simulink model "Multicopter_Testbed"  (R2012b)
settings: Solver=FixedStepDiscrete  SolverMode=SingleTasking  StartTime=0.0  StopTime=inf  FixedStep=Sampletime.Sim  MaxStep=0.005  MinStep=0.0001  RelTol=1e-5
PreLoadFcn:
  | addpath([cd filesep 'Multicopter_Simulation_Data'])
  | initMulticopterSimulationBus;
  | initOveroControlBus;
  | initMulticopterSimulation;
undefined symbols (not defined in the file): Airframe_Pelican, DiscIntNeverNeededParam, Environment_Earth, gcbh, quat_fr_euler, rad, Sampletime, Sensor_Autopilot, vrmfunc
(part 2 of 3)

== system Multicopter_Testbed/Ground_Control/Extended_Debug_Demux/Compare To Constant4 ==
  u : Inport
  Compare : RelationalOperator  Operator===  OutDataTypeStr=fixdt(0, 8)  ZeroCross=off  InputSameDT=on
  Constant : Constant  DisableCoverage=on  Value=const  OutDataTypeStr=Inherit: Inherit via back propagation
  y : Outport
  wires:
  u/1 -> Compare/1
  Constant/1 -> Compare/2
  Compare/1 -> y/1

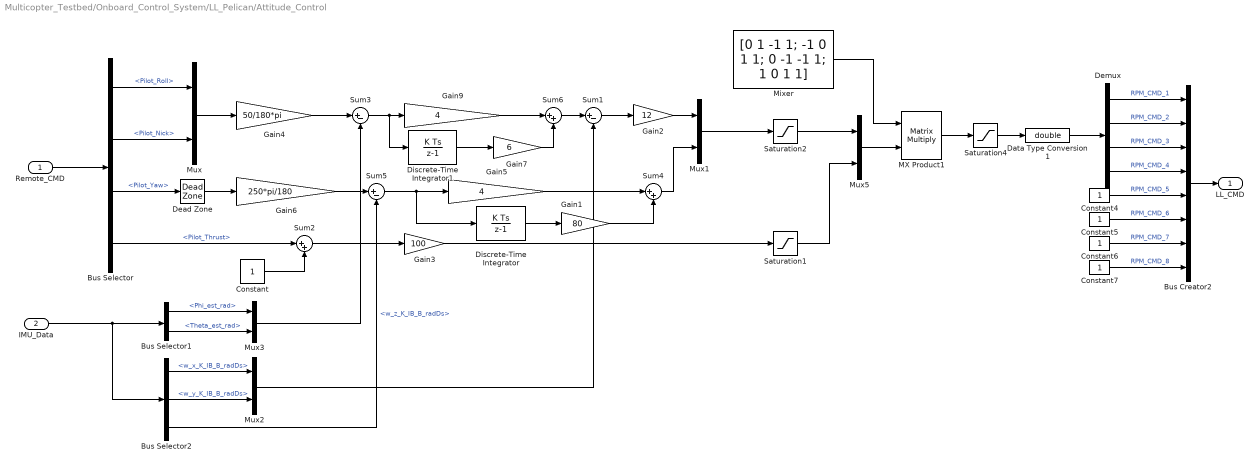
== system Multicopter_Testbed/Onboard_Control_System/LL_Pelican/Attitude_Control ==
  Remote_CMD : Inport
  IMU_Data : Inport  Port=2
  Bus Creator2 : BusCreator  Inputs=8
  Bus Selector : BusSelector  OutputSignals=Pilot_Roll,Pilot_Nick,Pilot_Yaw,Pilot_Thrust
  Bus Selector1 : BusSelector  OutputSignals=Phi_est_rad,Theta_est_rad
  Bus Selector2 : BusSelector  OutputSignals=w_x_K_IB_B_radDs,w_y_K_IB_B_radDs,w_z_K_IB_B_radDs
  Constant : Constant  OutDataTypeStr=single
  Constant{4..7} (4 alike) : Constant
  Data Type Conversion1 : DataTypeConversion  OutDataTypeStr=double
  Dead Zone : DeadZone  LowerValue=-0.1  UpperValue=0.1  SaturateOnIntegerOverflow=on
  Demux : Demux
  Discrete-Time Integrator : DiscreteIntegrator  SampleTime=-1  LimitOutput=on  UpperSaturationLimit=30/180*pi  LowerSaturationLimit=-30/180*pi  ICPrevOutput=DiscIntNeverNeededParam  ICPrevScaledInput=DiscIntNeverNeededParam
  Discrete-Time Integrator1 : DiscreteIntegrator  SampleTime=-1  LimitOutput=on  UpperSaturationLimit=5/180*pi  LowerSaturationLimit=-5/180*pi  ICPrevOutput=DiscIntNeverNeededParam  ICPrevScaledInput=DiscIntNeverNeededParam
  Gain1 : Gain  Gain=80
  Gain2 : Gain  Gain=12
  Gain3 : Gain  Gain=100
  Gain4 : Gain  Gain=50/180*pi
  Gain5 : Gain  Gain=4
  Gain6 : Gain  Gain=250*pi/180
  Gain7 : Gain  Gain=6
  Gain9 : Gain  Gain=4
  MX Product1 : Product  Multiplication=Matrix(*)  OutDataTypeStr=double  RndMeth=Simplest
  Mixer : Constant  Value=|  VectorParams1D=off  OutDataTypeStr=single
      | [0 1 -1 1; -1 0 1 1; 0 -1 -1 1;
      | 1 0 1 1]
  Mux{,1..3,5} (5 alike) : Mux  Inputs=2
  Saturation1 : Saturate  UpperLimit=170  LowerLimit=1
  Saturation2 : Saturate  UpperLimit=100  LowerLimit=-100
  Saturation4 : Saturate  UpperLimit=200  LowerLimit=1  OutDataTypeStr=int16
  Sum1 : Sum  Inputs=|+-
  Sum2 : Sum  Inputs=|++
  Sum3 : Sum  Inputs=|+-
  Sum4 : Sum  Inputs=|++
  Sum5 : Sum  Inputs=|+-
  Sum6 : Sum  Inputs=|++
  LL_CMD : Outport
  wires:
  Gain7/1 -> Sum6/2
  Discrete-Time Integrator1/1 -> Gain7/1
  Sum6/1 -> Sum1/1
  Data Type Conversion1/1 -> Demux/1
  Bus Creator2/1 -> LL_CMD/1
  Demux/4 -> Bus Creator2/4  "RPM_CMD_4"
  Demux/3 -> Bus Creator2/3  "RPM_CMD_3"
  Demux/2 -> Bus Creator2/2  "RPM_CMD_2"
  Demux/1 -> Bus Creator2/1  "RPM_CMD_1"
  Constant7/1 -> Bus Creator2/8  "RPM_CMD_8"
  Constant6/1 -> Bus Creator2/7  "RPM_CMD_7"
  Constant5/1 -> Bus Creator2/6  "RPM_CMD_6"
  Constant4/1 -> Bus Creator2/5  "RPM_CMD_5"
  Saturation4/1 -> Data Type Conversion1/1
  IMU_Data/1 -> Bus Selector2/1, Bus Selector1/1
  Gain4/1 -> Sum3/1
  Bus Selector1/2 -> Mux3/2  "<Theta_est_rad>"
  Bus Selector1/1 -> Mux3/1  "<Phi_est_rad>"
  Constant/1 -> Sum2/2
  Sum2/1 -> Gain3/1
  Saturation2/1 -> Mux5/1
  Saturation1/1 -> Mux5/2
  Mixer/1 -> MX Product1/1
  Mux5/1 -> MX Product1/2
  MX Product1/1 -> Saturation4/1
  Mux1/1 -> Saturation2/1
  Gain3/1 -> Saturation1/1
  Bus Selector/3 -> Dead Zone/1  "<Pilot_Yaw>"
  Bus Selector/2 -> Mux/2  "<Pilot_Nick>"
  Bus Selector/1 -> Mux/1  "<Pilot_Roll>"
  Remote_CMD/1 -> Bus Selector/1
  Mux3/1 -> Sum3/2
  Bus Selector2/3 -> Sum5/2  "<w_z_K_IB_B_radDs>"
  Mux/1 -> Gain4/1
  Bus Selector2/2 -> Mux2/2  "<w_y_K_IB_B_radDs>"
  Bus Selector2/1 -> Mux2/1  "<w_x_K_IB_B_radDs>"
  Sum3/1 -> Gain9/1, Discrete-Time Integrator1/1
  Bus Selector/4 -> Sum2/1  "<Pilot_Thrust>"
  Gain2/1 -> Mux1/1
  Sum5/1 -> Gain5/1, Discrete-Time Integrator/1
  Gain6/1 -> Sum5/1
  Sum1/1 -> Gain2/1
  Gain9/1 -> Sum6/1
  Mux2/1 -> Sum1/2
  Dead Zone/1 -> Gain6/1
  Discrete-Time Integrator/1 -> Gain1/1
  Gain1/1 -> Sum4/2
  Gain5/1 -> Sum4/1
  Sum4/1 -> Mux1/2

== system Multicopter_Testbed/Onboard_Control_System/LL_Pelican/Compare To Zero ==
  u : Inport
  Compare : RelationalOperator  Operator=>  OutDataTypeStr=fixdt(0, 8)  InputSameDT=on
  Constant : Constant  DisableCoverage=on  Value=0  OutDataTypeStr=Inherit: Inherit via back propagation  PreserveConstantTs=on
  y : Outport
  wires:
  Constant/1 -> Compare/2
  u/1 -> Compare/1
  Compare/1 -> y/1

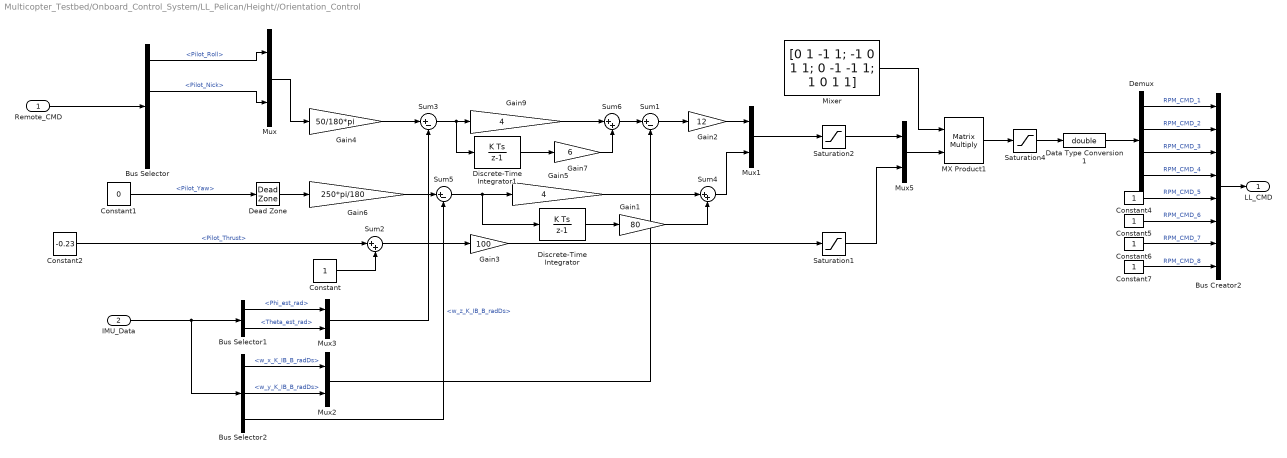
== system Multicopter_Testbed/Onboard_Control_System/LL_Pelican/Height//Orientation_Control ==
  Remote_CMD : Inport
  IMU_Data : Inport  Port=2
  Bus Creator2 : BusCreator  Inputs=8
  Bus Selector : BusSelector  OutputSignals=Pilot_Roll,Pilot_Nick,Pilot_Yaw,Pilot_Thrust
  Bus Selector1 : BusSelector  OutputSignals=Phi_est_rad,Theta_est_rad
  Bus Selector2 : BusSelector  OutputSignals=w_x_K_IB_B_radDs,w_y_K_IB_B_radDs,w_z_K_IB_B_radDs
  Constant : Constant  OutDataTypeStr=single
  Constant1 : Constant  Value=0  OutDataTypeStr=single
  Constant2 : Constant  Value=-0.23  OutDataTypeStr=single
  Constant{4..7} (4 alike) : Constant
  Data Type Conversion1 : DataTypeConversion  OutDataTypeStr=double
  Dead Zone : DeadZone  LowerValue=-0.1  UpperValue=0.1  SaturateOnIntegerOverflow=on
  Demux : Demux
  Discrete-Time Integrator : DiscreteIntegrator  SampleTime=-1  LimitOutput=on  UpperSaturationLimit=30/180*pi  LowerSaturationLimit=-30/180*pi  ICPrevOutput=DiscIntNeverNeededParam  ICPrevScaledInput=DiscIntNeverNeededParam
  Discrete-Time Integrator1 : DiscreteIntegrator  SampleTime=-1  LimitOutput=on  UpperSaturationLimit=5/180*pi  LowerSaturationLimit=-5/180*pi  ICPrevOutput=DiscIntNeverNeededParam  ICPrevScaledInput=DiscIntNeverNeededParam
  Gain1 : Gain  Gain=80
  Gain2 : Gain  Gain=12
  Gain3 : Gain  Gain=100
  Gain4 : Gain  Gain=50/180*pi
  Gain5 : Gain  Gain=4
  Gain6 : Gain  Gain=250*pi/180
  Gain7 : Gain  Gain=6
  Gain9 : Gain  Gain=4
  MX Product1 : Product  Multiplication=Matrix(*)  OutDataTypeStr=double  RndMeth=Simplest
  Mixer : Constant  Value=|  VectorParams1D=off  OutDataTypeStr=single
      | [0 1 -1 1; -1 0 1 1; 0 -1 -1 1;
      | 1 0 1 1]
  Mux{,1..3,5} (5 alike) : Mux  Inputs=2
  Saturation1 : Saturate  UpperLimit=170  LowerLimit=1
  Saturation2 : Saturate  UpperLimit=100  LowerLimit=-100
  Saturation4 : Saturate  UpperLimit=200  LowerLimit=1  OutDataTypeStr=int16
  Sum1 : Sum  Inputs=|+-
  Sum2 : Sum  Inputs=|++
  Sum3 : Sum  Inputs=|+-
  Sum4 : Sum  Inputs=|++
  Sum5 : Sum  Inputs=|+-
  Sum6 : Sum  Inputs=|++
  LL_CMD : Outport
  wires:
  Sum4/1 -> Mux1/2
  Gain5/1 -> Sum4/1
  Gain1/1 -> Sum4/2
  Discrete-Time Integrator/1 -> Gain1/1
  Dead Zone/1 -> Gain6/1
  Mux2/1 -> Sum1/2
  Gain9/1 -> Sum6/1
  Sum1/1 -> Gain2/1
  Gain6/1 -> Sum5/1
  Sum5/1 -> Discrete-Time Integrator/1, Gain5/1
  Gain2/1 -> Mux1/1
  Constant2/1 -> Sum2/1  "<Pilot_Thrust>"
  Sum3/1 -> Discrete-Time Integrator1/1, Gain9/1
  Bus Selector2/1 -> Mux2/1  "<w_x_K_IB_B_radDs>"
  Bus Selector2/2 -> Mux2/2  "<w_y_K_IB_B_radDs>"
  Mux/1 -> Gain4/1
  Bus Selector2/3 -> Sum5/2  "<w_z_K_IB_B_radDs>"
  Mux3/1 -> Sum3/2
  Remote_CMD/1 -> Bus Selector/1
  Bus Selector/1 -> Mux/1  "<Pilot_Roll>"
  Bus Selector/2 -> Mux/2  "<Pilot_Nick>"
  Constant1/1 -> Dead Zone/1  "<Pilot_Yaw>"
  Gain3/1 -> Saturation1/1
  Mux1/1 -> Saturation2/1
  MX Product1/1 -> Saturation4/1
  Mux5/1 -> MX Product1/2
  Mixer/1 -> MX Product1/1
  Saturation1/1 -> Mux5/2
  Saturation2/1 -> Mux5/1
  Sum2/1 -> Gain3/1
  Constant/1 -> Sum2/2
  Bus Selector1/1 -> Mux3/1  "<Phi_est_rad>"
  Bus Selector1/2 -> Mux3/2  "<Theta_est_rad>"
  Gain4/1 -> Sum3/1
  IMU_Data/1 -> Bus Selector1/1, Bus Selector2/1
  Saturation4/1 -> Data Type Conversion1/1
  Constant4/1 -> Bus Creator2/5  "RPM_CMD_5"
  Constant5/1 -> Bus Creator2/6  "RPM_CMD_6"
  Constant6/1 -> Bus Creator2/7  "RPM_CMD_7"
  Constant7/1 -> Bus Creator2/8  "RPM_CMD_8"
  Demux/1 -> Bus Creator2/1  "RPM_CMD_1"
  Demux/2 -> Bus Creator2/2  "RPM_CMD_2"
  Demux/3 -> Bus Creator2/3  "RPM_CMD_3"
  Demux/4 -> Bus Creator2/4  "RPM_CMD_4"
  Bus Creator2/1 -> LL_CMD/1
  Data Type Conversion1/1 -> Demux/1
  Sum6/1 -> Sum1/1
  Discrete-Time Integrator1/1 -> Gain7/1
  Gain7/1 -> Sum6/2

== system Multicopter_Testbed/Onboard_Control_System/LL_Signal_Processing/GPS_Signal_Processing ==
  Inputs : Inport  OutDataTypeStr=Bus: Sensor_Data_Bus
  Bus Creator1 : BusCreator  Inputs=16  OutDataTypeStr=Bus: FCS_GPS_Bus  NonVirtualBus=on
  Bus Selector : BusSelector  OutputSignals=GPS_Data.POS_lambda_WGS84,GPS_Data.POS_mue_WGS84,GPS_Data.POS_h_WGS84
  Bus Selector1 : BusSelector  OutputSignals=GPS_Data.VEL_x_E_O,GPS_Data.VEL_y_E_O
  Constant10 : Constant  Value=1696  OutDataTypeStr=int32
  Constant11 : Constant  Value=129600000  OutDataTypeStr=int32
  Constant12 : Constant  Value=6  OutDataTypeStr=int32
  Constant13 : Constant  Value=3  OutDataTypeStr=int32
  Constant14 : Constant  OutDataTypeStr=int32
  Constant15 : Constant  OutDataTypeStr=int32
  Constant5 : Constant  Value=0  OutDataTypeStr=single
  Constant6 : Constant  Value=8  OutDataTypeStr=single
  Constant7 : Constant  Value=15  OutDataTypeStr=single
  Constant8 : Constant  Value=1.2  OutDataTypeStr=single
  Constant9 : Constant  Value=60  OutDataTypeStr=single
  Gain1 : Gain  OutDataTypeStr=single  RndMeth=Simplest  LockScale=on
  Gain14 : Gain  OutDataTypeStr=double  RndMeth=Simplest  LockScale=on
  Gain15 : Gain  OutDataTypeStr=double  RndMeth=Simplest  LockScale=on
  Gain2 : Gain  OutDataTypeStr=single  RndMeth=Simplest  LockScale=on
  Gain3 : Gain  OutDataTypeStr=single  RndMeth=Simplest  LockScale=on
  Rate Transition{,1..4} (5 alike) : RateTransition  Integrity=off  OutPortSampleTime=Sampletime.Onboard
  GPS_Data : Outport  OutDataTypeStr=Bus: FCS_GPS_Bus
  wires:
  Rate Transition4/1 -> Gain2/1
  Rate Transition3/1 -> Gain1/1
  Rate Transition2/1 -> Gain3/1
  Rate Transition1/1 -> Gain15/1
  Rate Transition/1 -> Gain14/1
  Constant15/1 -> Bus Creator1/16  "diffS"
  Constant14/1 -> Bus Creator1/15  "flags"
  Gain2/1 -> Bus Creator1/5  "v_K_R_E_O_mDs"
  Gain1/1 -> Bus Creator1/4  "u_K_R_E_O_mDs"
  Gain3/1 -> Bus Creator1/3  "h_R_MSL_m"
  Gain15/1 -> Bus Creator1/2  "phi_R_WGS84_rad"
  Gain14/1 -> Bus Creator1/1  "lambda_R_WGS84_rad"
  Bus Selector/3 -> Rate Transition2/1  "<POS_h_WGS84>"
  Bus Selector/2 -> Rate Transition1/1  "<POS_mue_WGS84>"
  Bus Selector/1 -> Rate Transition/1  "<POS_lambda_WGS84>"
  Constant13/1 -> Bus Creator1/14  "fixtype"
  Constant12/1 -> Bus Creator1/13  "num_sv"
  Constant11/1 -> Bus Creator1/12  "time_of_week_ms"
  Constant10/1 -> Bus Creator1/11  "week_1"
  Constant9/1 -> Bus Creator1/7  "chi_K_rad"
  Constant8/1 -> Bus Creator1/10  "accuracy_speed_mDs"
  Constant7/1 -> Bus Creator1/9  "accuracy_vertical_m"
  Constant6/1 -> Bus Creator1/8  "accuracy_horizontal_m"
  Constant5/1 -> Bus Creator1/6  "w_K_R_E_O_mDs"
  Bus Creator1/1 -> GPS_Data/1
  Inputs/1 -> Bus Selector1/1, Bus Selector/1
  Bus Selector1/1 -> Rate Transition3/1  "<VEL_x_E_O>"
  Bus Selector1/2 -> Rate Transition4/1  "<VEL_y_E_O>"

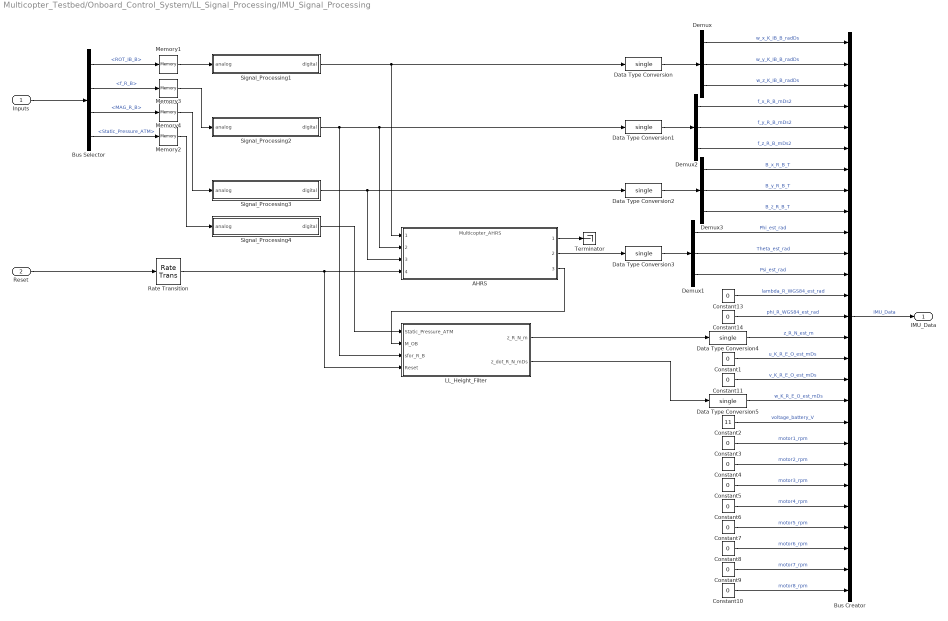
== system Multicopter_Testbed/Onboard_Control_System/LL_Signal_Processing/IMU_Signal_Processing ==
  Inputs : Inport  OutDataTypeStr=Bus: Sensor_Data_Bus
  Reset : Inport  Port=2
  AHRS : ModelReference  ModelNameDialog=Multicopter_AHRS  ModelReferenceVersion=1.8  CopyOfModelName=Multicopter_AHRS  CopyOfModelProtected=on  DefaultDataLogging=off
  Bus Creator : BusCreator  Inputs=27  OutDataTypeStr=Bus: FCS_IMU_Bus  NonVirtualBus=on
  Bus Selector : BusSelector  OutputSignals=ROT_IB_B,f_R_B,MAG_R_B,Static_Pressure_ATM
  Constant1 : Constant  Value=0  OutDataTypeStr=single
  Constant{3..10} (8 alike) : Constant  Value=0  OutDataTypeStr=int32
  Constant11 : Constant  Value=0  OutDataTypeStr=single
  Constant13 : Constant  Value=0  OutDataTypeStr=double
  Constant14 : Constant  Value=0  OutDataTypeStr=double
  Constant2 : Constant  Value=11  OutDataTypeStr=single
  Data Type Conversion{,1..5} (6 alike) : DataTypeConversion  OutDataTypeStr=single
  Demux{,1..3} (4 alike) : Demux  Outputs=3
  LL_Height_Filter : Subsystem
  Memory{1..4} (4 alike) : Memory  InheritSampleTime=on
  Rate Transition : RateTransition  Integrity=off  OutPortSampleTime=Sampletime.Onboard
  Signal_Processing1 : Subsystem  mask{Sensor=Sensor_Autopilot.ROT}
      mask prompts: Sensor "Sensor Data"
  Signal_Processing2 : Subsystem  mask{Sensor=Sensor_Autopilot.ACC}
      mask prompts: Sensor "Sensor Data"
  Signal_Processing3 : Subsystem  mask{Sensor=Sensor_Autopilot.MAG}
      mask prompts: Sensor "Sensor Data"
  Signal_Processing4 : Subsystem  mask{Sensor=Sensor_Autopilot.BARO}
      mask prompts: Sensor "Sensor Data"
  Terminator : Terminator
  IMU_Data : Outport  OutDataTypeStr=Bus: FCS_IMU_Bus
  wires:
  Data Type Conversion3/1 -> Demux1/1
  Data Type Conversion2/1 -> Demux3/1
  Data Type Conversion1/1 -> Demux2/1
  Data Type Conversion/1 -> Demux/1
  Memory4/1 -> Signal_Processing3/1(analog)
  Demux3/3 -> Bus Creator/9  "B_z_R_B_T"
  Demux3/2 -> Bus Creator/8  "B_y_R_B_T"
  Demux3/1 -> Bus Creator/7  "B_x_R_B_T"
  Memory3/1 -> Signal_Processing2/1(analog)
  Memory1/1 -> Signal_Processing1/1(analog)
  Demux2/3 -> Bus Creator/6  "f_z_R_B_mDs2"
  Demux2/2 -> Bus Creator/5  "f_y_R_B_mDs2"
  Demux2/1 -> Bus Creator/4  "f_x_R_B_mDs2"
  Demux1/3 -> Bus Creator/12  "Psi_est_rad"
  Demux1/2 -> Bus Creator/11  "Theta_est_rad"
  Demux1/1 -> Bus Creator/10  "Phi_est_rad"
  Demux/3 -> Bus Creator/3  "w_z_K_IB_B_radDs"
  Demux/2 -> Bus Creator/2  "w_y_K_IB_B_radDs"
  Demux/1 -> Bus Creator/1  "w_x_K_IB_B_radDs"
  Inputs/1 -> Bus Selector/1
  Signal_Processing1/1(digital) -> AHRS/1, Data Type Conversion/1
  Signal_Processing2/1(digital) -> AHRS/2, Data Type Conversion1/1, LL_Height_Filter/3(sfor_R_B)
  Signal_Processing3/1(digital) -> AHRS/3, Data Type Conversion2/1
  Bus Selector/2 -> Memory3/1  "<f_R_B>"
  Bus Selector/1 -> Memory1/1  "<ROT_IB_B>"
  Bus Selector/3 -> Memory4/1  "<MAG_R_B>"
  Bus Creator/1 -> IMU_Data/1  "IMU_Data"
  LL_Height_Filter/1(z_R_N_m) -> Data Type Conversion4/1
  LL_Height_Filter/2(z_dot_R_N_mDs) -> Data Type Conversion5/1
  Bus Selector/4 -> Memory2/1  "<Static_Pressure_ATM>"
  Signal_Processing4/1(digital) -> LL_Height_Filter/1(Static_Pressure_ATM)
  Memory2/1 -> Signal_Processing4/1(analog)
  Data Type Conversion4/1 -> Bus Creator/15  "z_R_N_est_m"
  Data Type Conversion5/1 -> Bus Creator/18  "w_K_R_E_O_est_mDs"
  Constant10/1 -> Bus Creator/27  "motor8_rpm"
  Constant9/1 -> Bus Creator/26  "motor7_rpm"
  Constant8/1 -> Bus Creator/25  "motor6_rpm"
  Constant7/1 -> Bus Creator/24  "motor5_rpm"
  Constant6/1 -> Bus Creator/23  "motor4_rpm"
  Constant5/1 -> Bus Creator/22  "motor3_rpm"
  Constant4/1 -> Bus Creator/21  "motor2_rpm"
  Constant3/1 -> Bus Creator/20  "motor1_rpm"
  Constant2/1 -> Bus Creator/19  "voltage_battery_V"
  Constant1/1 -> Bus Creator/16  "u_K_R_E_O_est_mDs"
  Constant11/1 -> Bus Creator/17  "v_K_R_E_O_est_mDs"
  Constant14/1 -> Bus Creator/14  "phi_R_WGS84_est_rad"
  Constant13/1 -> Bus Creator/13  "lambda_R_WGS84_est_rad"
  AHRS/3 -> LL_Height_Filter/2(M_OB)
  Reset/1 -> Rate Transition/1
  Rate Transition/1 -> LL_Height_Filter/4(Reset), AHRS/4
  AHRS/1 -> Terminator/1
  AHRS/2 -> Data Type Conversion3/1

== system Multicopter_Testbed/Onboard_Control_System/LL_Signal_Processing/RC_Signal_Processing ==
  Remote : Inport
  Bus Creator : BusCreator  Inputs=7  OutDataTypeStr=Bus: FCS_Pilot_Bus  NonVirtualBus=on
  Demux1 : Demux  Outputs=7
  Gain : Gain  Gain=2^7  OutDataTypeStr=int16  RndMeth=Simplest
  Gain1 : Gain  Gain=2^-7  OutDataTypeStr=single  RndMeth=Simplest
  Rate Transition2 : RateTransition  Integrity=off  OutPortSampleTime=Sampletime.Onboard*10
  RC_Data : Outport  OutDataTypeStr=Bus: FCS_Pilot_Bus
  wires:
  Bus Creator/1 -> RC_Data/1
  Demux1/7 -> Bus Creator/7  "Pilot_Gain"
  Demux1/6 -> Bus Creator/6  "Pilot_SW_Mode"
  Demux1/5 -> Bus Creator/5  "Pilot_SW_HL"
  Demux1/4 -> Bus Creator/4  "Pilot_Thrust"
  Demux1/3 -> Bus Creator/3  "Pilot_Yaw"
  Demux1/2 -> Bus Creator/2  "Pilot_Nick"
  Demux1/1 -> Bus Creator/1  "Pilot_Roll"
  Remote/1 -> Gain/1
  Gain/1 -> Gain1/1
  Rate Transition2/1 -> Demux1/1
  Gain1/1 -> Rate Transition2/1

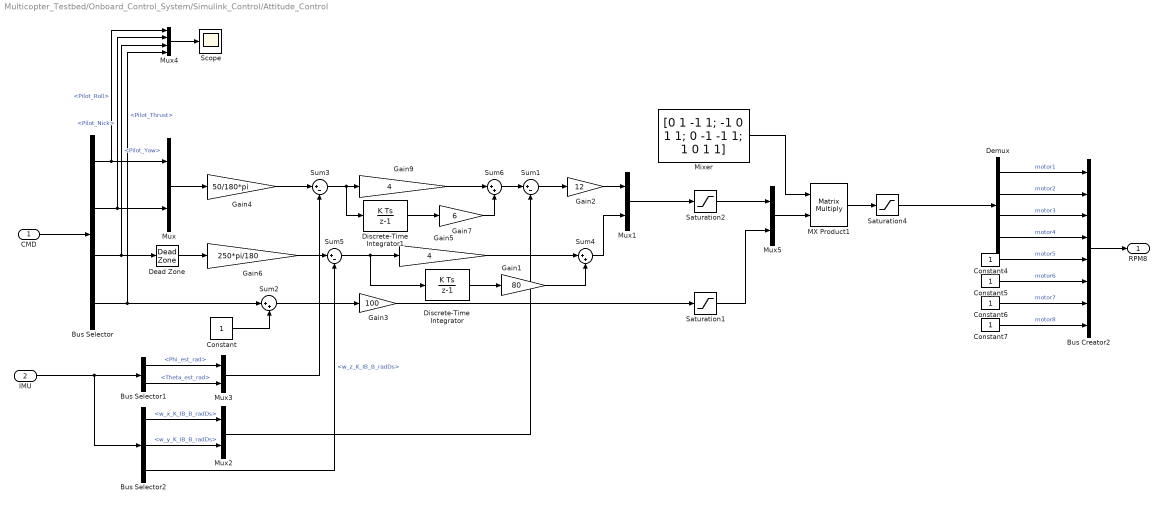
== system Multicopter_Testbed/Onboard_Control_System/Simulink_Control/Attitude_Control ==
  CMD : Inport
  IMU : Inport  Port=2
  Bus Creator2 : BusCreator  Inputs=8
  Bus Selector : BusSelector  OutputSignals=Pilot_Roll,Pilot_Nick,Pilot_Yaw,Pilot_Thrust
  Bus Selector1 : BusSelector  OutputSignals=Phi_est_rad,Theta_est_rad
  Bus Selector2 : BusSelector  OutputSignals=w_x_K_IB_B_radDs,w_y_K_IB_B_radDs,w_z_K_IB_B_radDs
  Constant : Constant  OutDataTypeStr=single
  Constant{4..7} (4 alike) : Constant  OutDataTypeStr=int16
  Dead Zone : DeadZone  LowerValue=-0.1  UpperValue=0.1  SaturateOnIntegerOverflow=on
  Demux : Demux
  Discrete-Time Integrator : DiscreteIntegrator  SampleTime=-1  LimitOutput=on  UpperSaturationLimit=30/180*pi  LowerSaturationLimit=-30/180*pi  ICPrevOutput=DiscIntNeverNeededParam  ICPrevScaledInput=DiscIntNeverNeededParam
  Discrete-Time Integrator1 : DiscreteIntegrator  SampleTime=-1  LimitOutput=on  UpperSaturationLimit=5/180*pi  LowerSaturationLimit=-5/180*pi  ICPrevOutput=DiscIntNeverNeededParam  ICPrevScaledInput=DiscIntNeverNeededParam
  Gain1 : Gain  Gain=80
  Gain2 : Gain  Gain=12
  Gain3 : Gain  Gain=100
  Gain4 : Gain  Gain=50/180*pi
  Gain5 : Gain  Gain=4
  Gain6 : Gain  Gain=250*pi/180
  Gain7 : Gain  Gain=6
  Gain9 : Gain  Gain=4
  MX Product1 : Product  Multiplication=Matrix(*)  OutDataTypeStr=double  RndMeth=Simplest
  Mixer : Constant  Value=|  VectorParams1D=off  OutDataTypeStr=single
      | [0 1 -1 1; -1 0 1 1; 0 -1 -1 1;
      | 1 0 1 1]
  Mux{,1..3,5} (5 alike) : Mux  Inputs=2
  Mux4 : Mux
  Saturation1 : Saturate  UpperLimit=170  LowerLimit=1
  Saturation2 : Saturate  UpperLimit=100  LowerLimit=-100
  Saturation4 : Saturate  UpperLimit=200  LowerLimit=1  OutDataTypeStr=int16
  Scope : Scope
      settings: ShowLegends=on  TimeRange=10  YMin=-0.35  YMax=0  SaveName=ScopeData14
  Sum1 : Sum  Inputs=|+-
  Sum2 : Sum  Inputs=|++
  Sum3 : Sum  Inputs=|+-
  Sum4 : Sum  Inputs=|++
  Sum5 : Sum  Inputs=|+-
  Sum6 : Sum  Inputs=|++
  RPM8 : Outport
  wires:
  Gain7/1 -> Sum6/2
  Discrete-Time Integrator1/1 -> Gain7/1
  Sum6/1 -> Sum1/1
  Demux/4 -> Bus Creator2/4  "motor4"
  Demux/3 -> Bus Creator2/3  "motor3"
  Demux/2 -> Bus Creator2/2  "motor2"
  Demux/1 -> Bus Creator2/1  "motor1"
  Constant7/1 -> Bus Creator2/8  "motor8"
  Constant6/1 -> Bus Creator2/7  "motor7"
  Constant5/1 -> Bus Creator2/6  "motor6"
  Constant4/1 -> Bus Creator2/5  "motor5"
  Saturation4/1 -> Demux/1
  IMU/1 -> Bus Selector2/1, Bus Selector1/1
  Gain4/1 -> Sum3/1
  Bus Selector1/2 -> Mux3/2  "<Theta_est_rad>"
  Bus Selector1/1 -> Mux3/1  "<Phi_est_rad>"
  Constant/1 -> Sum2/2
  Sum2/1 -> Gain3/1
  Saturation2/1 -> Mux5/1
  Saturation1/1 -> Mux5/2
  Mixer/1 -> MX Product1/1
  Mux5/1 -> MX Product1/2
  MX Product1/1 -> Saturation4/1
  Mux1/1 -> Saturation2/1
  Gain3/1 -> Saturation1/1
  Bus Selector/3 -> Mux4/3, Dead Zone/1  "<Pilot_Yaw>"
  Bus Selector/2 -> Mux4/2, Mux/2  "<Pilot_Nick>"
  Bus Selector/1 -> Mux4/1, Mux/1  "<Pilot_Roll>"
  CMD/1 -> Bus Selector/1
  Mux3/1 -> Sum3/2
  Bus Selector2/3 -> Sum5/2  "<w_z_K_IB_B_radDs>"
  Mux/1 -> Gain4/1
  Bus Selector2/2 -> Mux2/2  "<w_y_K_IB_B_radDs>"
  Bus Selector2/1 -> Mux2/1  "<w_x_K_IB_B_radDs>"
  Sum3/1 -> Gain9/1, Discrete-Time Integrator1/1
  Bus Selector/4 -> Mux4/4, Sum2/1  "<Pilot_Thrust>"
  Gain2/1 -> Mux1/1
  Sum5/1 -> Gain5/1, Discrete-Time Integrator/1
  Gain6/1 -> Sum5/1
  Sum1/1 -> Gain2/1
  Gain9/1 -> Sum6/1
  Mux2/1 -> Sum1/2
  Dead Zone/1 -> Gain6/1
  Discrete-Time Integrator/1 -> Gain1/1
  Gain1/1 -> Sum4/2
  Gain5/1 -> Sum4/1
  Sum4/1 -> Mux1/2
  Bus Creator2/1 -> RPM8/1
  Mux4/1 -> Scope/1

== system Multicopter_Testbed/Onboard_Control_System/Simulink_Control/CMD_Mapping_Quadcopter ==
  note: Hummingbird/Pelican Mapping
  note: Direct individual motor control (range: 0..200 = 0..100 %)
      |
      | Quadcopter (AscTec Hummingbird, AscTec Pelican):
      |  * motor_1: front
      |  * motor_2: rear
      |  * motor_3: left
      |  * motor_4: right
      |
      | Hexcopter (AscTec Firefly):
      |  * motor_1: front-left
      |  * motor_2: left
      |  * motor_3: rear-left
      |  * motor_4: rear-right
      |  * motor_5: right
      |  * motor_6: front-right
  RPM8_CMD : Inport
  Enable_Flag : Inport  Port=2
  Bus Creator : BusCreator  Inputs=10  OutDataTypeStr=Bus: FCS_CMD_Bus  NonVirtualBus=on
  Bus Selector : BusSelector  OutputSignals=motor1,motor2,motor3 ,motor4,motor5,motor6,motor7,motor8
  Constant12 : Constant  Value=0  OutDataTypeStr=int16
  Data Type Conversion : DataTypeConversion  OutDataTypeStr=int16
  HL_CMD : Outport  OutDataTypeStr=Bus: FCS_CMD_Bus  BusOutputAsStruct=on
  wires:
  Data Type Conversion/1 -> Bus Creator/9  "mode"
  Constant12/1 -> Bus Creator/10  "heartbeat"
  Enable_Flag/1 -> Data Type Conversion/1
  Bus Creator/1 -> HL_CMD/1
  RPM8_CMD/1 -> Bus Selector/1
  Bus Selector/1 -> Bus Creator/1  "<motor1>"
  Bus Selector/2 -> Bus Creator/2  "<motor2>"
  Bus Selector/3 -> Bus Creator/3  "<motor3 >"
  Bus Selector/4 -> Bus Creator/4  "<motor4>"
  Bus Selector/5 -> Bus Creator/5  "<motor5>"
  Bus Selector/6 -> Bus Creator/6  "<motor6>"
  Bus Selector/7 -> Bus Creator/7  "<motor7>"
  Bus Selector/8 -> Bus Creator/8  "<motor8>"

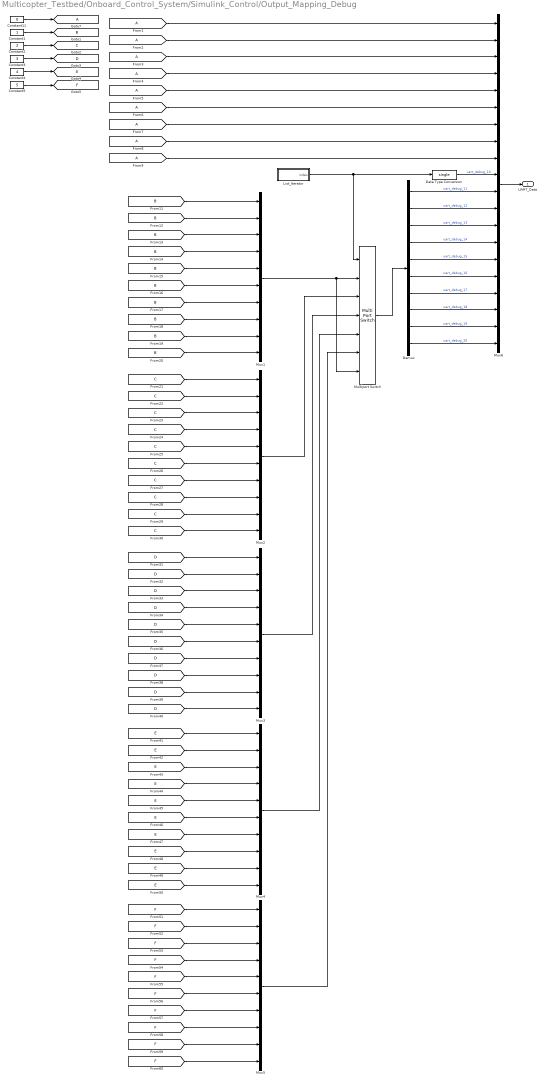
== system Multicopter_Testbed/Onboard_Control_System/Simulink_Control/Output_Mapping_Debug ==
  Constant1 : Constant  OutDataTypeStr=single
  Constant11 : Constant  Value=0  OutDataTypeStr=single
  Constant2 : Constant  Value=2  OutDataTypeStr=single
  Constant3 : Constant  Value=3  OutDataTypeStr=single
  Constant4 : Constant  Value=4  OutDataTypeStr=single
  Constant5 : Constant  Value=5  OutDataTypeStr=single
  Data Type Conversion : DataTypeConversion  OutDataTypeStr=single
  Demux : Demux  Outputs=10
  List_Iterator : Subsystem  mask(Iterator){list=[1;2;3;4;5;], dec=1}
      mask prompts: list "List of indices to iterate"; dec "Rate decimation"
      mask help: Outputs a sequence of numbers specified by a list of arbitrary length. The rate can be decimated by an integer factor.
  Multiport Switch : MultiPortSwitch  Inputs=5  DataPortForDefault=Additional data port  DiagnosticForDefault=None  InputSameDT=on
  Mux{1..5} (5 alike) : Mux  Inputs=10
  Mux6 : Mux  Inputs=20
  UART_Data : Outport
  tag scope: A=global, B=global, C=global, D=global, E=global, F=global
  wires:
  Data Type Conversion/1 -> Mux6/10  "uart_debug_10"
  Mux6/1 -> UART_Data/1
  Demux/1 -> Mux6/11  "uart_debug_11"
  Demux/2 -> Mux6/12  "uart_debug_12"
  Demux/3 -> Mux6/13  "uart_debug_13"
  Demux/4 -> Mux6/14  "uart_debug_14"
  Demux/5 -> Mux6/15  "uart_debug_15"
  Demux/6 -> Mux6/16  "uart_debug_16"
  Demux/7 -> Mux6/17  "uart_debug_17"
  Demux/8 -> Mux6/18  "uart_debug_18"
  Demux/9 -> Mux6/19  "uart_debug_19"
  Demux/10 -> Mux6/20  "uart_debug_20"
  [A] -> Mux6/1
  [A] -> Mux6/2
  [A] -> Mux6/3
  [A] -> Mux6/4
  [A] -> Mux6/5
  [A] -> Mux6/6
  [A] -> Mux6/7
  [A] -> Mux6/8
  [A] -> Mux6/9
  [B] -> Mux1/1
  [B] -> Mux1/2
  [B] -> Mux1/3
  [B] -> Mux1/4
  [B] -> Mux1/5
  [B] -> Mux1/6
  [B] -> Mux1/7
  [B] -> Mux1/8
  [B] -> Mux1/9
  [B] -> Mux1/10
  Mux1/1 -> Multiport Switch/2, Multiport Switch/7
  [C] -> Mux2/1
  [C] -> Mux2/2
  [C] -> Mux2/3
  [C] -> Mux2/4
  [C] -> Mux2/5
  [C] -> Mux2/6
  [C] -> Mux2/7
  [C] -> Mux2/8
  [C] -> Mux2/9
  [C] -> Mux2/10
  Mux2/1 -> Multiport Switch/3
  [D] -> Mux3/1
  [D] -> Mux3/2
  [D] -> Mux3/3
  [D] -> Mux3/4
  [D] -> Mux3/5
  [D] -> Mux3/6
  [D] -> Mux3/7
  [D] -> Mux3/8
  [D] -> Mux3/9
  [D] -> Mux3/10
  Mux3/1 -> Multiport Switch/4
  [E] -> Mux4/1
  [E] -> Mux4/2
  [E] -> Mux4/3
  [E] -> Mux4/4
  [E] -> Mux4/5
  [E] -> Mux4/6
  [E] -> Mux4/7
  [E] -> Mux4/8
  [E] -> Mux4/9
  [E] -> Mux4/10
  Mux4/1 -> Multiport Switch/5
  Multiport Switch/1 -> Demux/1
  [F] -> Mux5/1
  [F] -> Mux5/2
  [F] -> Mux5/3
  [F] -> Mux5/4
  [F] -> Mux5/5
  [F] -> Mux5/6
  [F] -> Mux5/7
  [F] -> Mux5/8
  [F] -> Mux5/9
  [F] -> Mux5/10
  Mux5/1 -> Multiport Switch/6
  List_Iterator/1(index) -> Data Type Conversion/1, Multiport Switch/1
  Constant11/1 -> [A]
  Constant1/1 -> [B]
  Constant2/1 -> [C]
  Constant3/1 -> [D]
  Constant4/1 -> [E]
  Constant5/1 -> [F]

== system Multicopter_Testbed/Vision_dummy/Attitude Estimation/ADC1 ==
  analog : Inport
  Constant : Constant  Value=resolution
  Divide : Product  Inputs=*/  OutDataTypeStr=int32
  Product : Product  OutDataTypeStr=double  RndMeth=Zero
  digital : Outport
  wires:
  Constant/1 -> Product/2, Divide/2
  analog/1 -> Divide/1
  Divide/1 -> Product/1
  Product/1 -> digital/1

== system Multicopter_Testbed/Vision_dummy/Attitude Estimation/Euler to Quat ==
  euler : Inport
  Add : Sum
  Add1 : Sum  Inputs=+-
  Add2 : Sum
  Add3 : Sum  Inputs=+-
  Demux : Demux  Outputs=3
  Gain : Gain  Gain=0.5
  Matrix Concatenate : Concatenate  NumInputs=4  ConcatenateDimension=2
  Product{,1..7} (8 alike) : Product  Inputs=3  RndMeth=Zero
  Trigonometric Function : Trigonometry
  Trigonometric Function1 : Trigonometry  Operator=cos
  Trigonometric Function2 : Trigonometry
  Trigonometric Function3 : Trigonometry  Operator=cos
  Trigonometric Function4 : Trigonometry
  Trigonometric Function5 : Trigonometry  Operator=cos
  q : Outport
  wires:
  euler/1 -> Gain/1
  Gain/1 -> Demux/1
  Demux/3 -> Trigonometric Function4/1, Trigonometric Function5/1  "psi"
  Demux/2 -> Trigonometric Function2/1, Trigonometric Function3/1  "theta"
  Demux/1 -> Trigonometric Function/1, Trigonometric Function1/1  "phi"
  Product/1 -> Add/1
  Product1/1 -> Add/2
  Product2/1 -> Add1/1
  Product3/1 -> Add1/2
  Product4/1 -> Add2/1
  Product5/1 -> Add2/2
  Product6/1 -> Add3/1
  Product7/1 -> Add3/2
  Add/1 -> Matrix Concatenate/1
  Add1/1 -> Matrix Concatenate/2
  Add2/1 -> Matrix Concatenate/3
  Add3/1 -> Matrix Concatenate/4
  Matrix Concatenate/1 -> q/1
  Trigonometric Function5/1 -> Product7/3, Product4/3, Product2/3, Product/3  "c_ps"
  Trigonometric Function2/1 -> Product7/2, Product4/2, Product3/2, Product1/2  "s_th"
  Trigonometric Function/1 -> Product7/1, Product5/1, Product2/1, Product1/1  "s_ph"
  Trigonometric Function4/1 -> Product6/3, Product5/3, Product3/3, Product1/3  "s_ps"
  Trigonometric Function3/1 -> Product6/2, Product5/2, Product2/2, Product/2  "c_th"
  Trigonometric Function1/1 -> Product6/1, Product4/1, Product3/1, Product/1  "c_ph"

== system Multicopter_Testbed/Vision_dummy/Attitude Estimation/Gauss Markow ==
  Add : Sum
  Add1 : Sum
  Gain : Gain  Gain=sigma.*sqrt (2./t_corr)
  Gain1 : Gain  Gain=-1./t_corr
  Gain2 : Gain  Gain=T_s
  Memory : Memory  InheritSampleTime=on
  Random Number : RandomNumber  Mean=zeros(dim,1)  Variance=ones(dim, 1)  Seed=floor(rand(dim, 1).*123456)  SampleTime=T_s  VectorParams1D=off
  Noise : Outport  PortDimensions=3
  wires:
  Memory/1 -> Gain1/1, Add1/1
  Random Number/1 -> Gain/1
  Gain/1 -> Add/2
  Gain1/1 -> Add/1
  Add/1 -> Gain2/1  "w_dot"
  Gain2/1 -> Add1/2
  Add1/1 -> Memory/1, Noise/1  "w"

== system Multicopter_Testbed/Vision_dummy/Attitude Estimation/Quat to Euler ==
  q : Inport
  Add : Sum  Inputs=++--
  Add1 : Sum
  Add2 : Sum  Inputs=+-
  Add4 : Sum
  Add8 : Sum  Inputs=+--+
  Constant : Constant  OutDataTypeStr=Inherit: Inherit via back propagation
  Constant1 : Constant  Value=-1  OutDataTypeStr=Inherit: Inherit via back propagation
  Data Type Duplicate : DataTypeDuplicate  NumInputPorts=4
  Demux1 : Demux
  Demux2 : Demux
  Gain : Gain  Gain=2  OutDataTypeStr=Inherit: Same as input
  Gain1 : Gain  Gain=-2  OutDataTypeStr=Inherit: Same as input
  Gain3 : Gain  Gain=2  OutDataTypeStr=Inherit: Same as input
  Max : MinMax  Function=max  Inputs=2
  Min : MinMax  Inputs=2
  Mux : Mux  Inputs=3
  Product{,1..4,7..8} (7 alike) : Product  RndMeth=Zero
  Trigonometric Function1 : Trigonometry  Operator=atan2  OutputSignalType=real
  Trigonometric Function2 : Trigonometry  Operator=asin  OutputSignalType=real
  Trigonometric Function6 : Trigonometry  Operator=atan2  OutputSignalType=real
  euler : Outport
  wires:
  Constant1/1 -> Max/2
  Min/1 -> Max/1
  Constant/1 -> Min/2
  Gain1/1 -> Min/1
  Max/1 -> Trigonometric Function2/1
  Demux1/2 -> Product8/2, Product3/1, Product1/1  "q2"
  Add8/1 -> Trigonometric Function6/2
  Gain3/1 -> Trigonometric Function6/1
  Product8/1 -> Add4/2
  Product7/1 -> Add4/1
  Add4/1 -> Gain3/1
  Product4/1 -> Add2/2
  Product3/1 -> Add2/1
  Add2/1 -> Gain1/1
  Product2/1 -> Add1/2
  Product1/1 -> Add1/1
  Gain/1 -> Trigonometric Function1/1
  Add1/1 -> Gain/1
  Add/1 -> Trigonometric Function1/2
  Demux1/1 -> Product8/1, Product4/1, Product2/1  "q1"
  Demux1/3 -> Product7/1, Product4/2, Product1/2  "q3"
  Demux1/4 -> Product7/2, Product3/2, Product2/2  "q4"
  Demux2/4 -> Add8/4, Add/4  "q4^2"
  Demux2/3 -> Add8/3, Add/3  "q3^2"
  Demux2/2 -> Add8/2, Add/2  "q2^2"
  Demux2/1 -> Add8/1, Add/1  "q1^2"
  Product/1 -> Demux2/1
  Trigonometric Function2/1 -> Mux/2, Data Type Duplicate/3
  Trigonometric Function1/1 -> Mux/3, Data Type Duplicate/4
  Trigonometric Function6/1 -> Mux/1, Data Type Duplicate/2
  Mux/1 -> euler/1
  q/1 -> Product/2, Product/1, Demux1/1, Data Type Duplicate/1

== system Multicopter_Testbed/Vision_dummy/Position Estimation/ADC1 ==
  analog : Inport
  Constant : Constant  Value=resolution
  Divide : Product  Inputs=*/  OutDataTypeStr=int32
  Product : Product  OutDataTypeStr=double  RndMeth=Zero
  digital : Outport
  wires:
  Constant/1 -> Product/2, Divide/2
  analog/1 -> Divide/1
  Divide/1 -> Product/1
  Product/1 -> digital/1

== system Multicopter_Testbed/Vision_dummy/Position Estimation/Gauss Markow1 ==
  Add : Sum
  Add1 : Sum
  Gain : Gain  Gain=sigma.*sqrt (2./t_corr)
  Gain1 : Gain  Gain=-1./t_corr
  Gain2 : Gain  Gain=T_s
  Memory : Memory  InheritSampleTime=on
  Random Number : RandomNumber  Mean=zeros(dim,1)  Variance=ones(dim, 1)  Seed=floor(rand(dim, 1).*123456)  SampleTime=T_s  VectorParams1D=off
  Noise : Outport  PortDimensions=3
  wires:
  Memory/1 -> Gain1/1, Add1/1
  Random Number/1 -> Gain/1
  Gain/1 -> Add/2
  Gain1/1 -> Add/1
  Add/1 -> Gain2/1  "w_dot"
  Gain2/1 -> Add1/2
  Add1/1 -> Memory/1, Noise/1  "w"

== system Multicopter_Testbed/Visualisation/Propulsion_System/RPM_Mapping ==
  MOT_CMD : Inport
  Constant : Constant  Value=0
  Gain1 : Gain  DisableCoverage=on  Gain=n_max-n_min  SaturateOnIntegerOverflow=on  OutDataTypeStr=Inherit: Same as input
  Gain3 : Gain  Gain=2*pi/60
  Gain4 : Gain  DisableCoverage=on  Gain=n_min  OutDataTypeStr=Inherit: Inherit via back propagation  SaturateOnIntegerOverflow=on
  Sign : Signum  DisableCoverage=on
  Sum1 : Sum  Inputs=|++  SaturateOnIntegerOverflow=on  InputSameDT=on  OutDataTypeStr=Inherit: Same as first input
  Switch : Switch  Criteria=u2 ~= 0
  ROT_CMD : Outport
  wires:
  Sum1/1 -> Gain3/1
  Gain1/1 -> Sum1/2
  Gain4/1 -> Sum1/1
  Sign/1 -> Gain4/1
  Switch/1 -> ROT_CMD/1
  Gain3/1 -> Switch/1
  Constant/1 -> Switch/3
  MOT_CMD/1 -> Gain1/1, Sign/1, Switch/2

== system Multicopter_Testbed/Visualisation/Propulsion_System/RPM_Mapping1 ==
  MOT_CMD : Inport
  Constant : Constant  Value=0
  Gain1 : Gain  DisableCoverage=on  Gain=n_max-n_min  SaturateOnIntegerOverflow=on  OutDataTypeStr=Inherit: Same as input
  Gain3 : Gain  Gain=2*pi/60
  Gain4 : Gain  DisableCoverage=on  Gain=n_min  OutDataTypeStr=Inherit: Inherit via back propagation  SaturateOnIntegerOverflow=on
  Sign : Signum  DisableCoverage=on
  Sum1 : Sum  Inputs=|++  SaturateOnIntegerOverflow=on  InputSameDT=on  OutDataTypeStr=Inherit: Same as first input
  Switch : Switch  Criteria=u2 ~= 0
  ROT_CMD : Outport
  wires:
  MOT_CMD/1 -> Switch/2, Sign/1, Gain1/1
  Constant/1 -> Switch/3
  Gain3/1 -> Switch/1
  Switch/1 -> ROT_CMD/1
  Sign/1 -> Gain4/1
  Gain4/1 -> Sum1/1
  Gain1/1 -> Sum1/2
  Sum1/1 -> Gain3/1

== system Multicopter_Testbed/Visualisation/Propulsion_System/RPM_Mapping2 ==
  MOT_CMD : Inport
  Constant : Constant  Value=0
  Gain1 : Gain  DisableCoverage=on  Gain=n_max-n_min  SaturateOnIntegerOverflow=on  OutDataTypeStr=Inherit: Same as input
  Gain3 : Gain  Gain=2*pi/60
  Gain4 : Gain  DisableCoverage=on  Gain=n_min  OutDataTypeStr=Inherit: Inherit via back propagation  SaturateOnIntegerOverflow=on
  Sign : Signum  DisableCoverage=on
  Sum1 : Sum  Inputs=|++  SaturateOnIntegerOverflow=on  InputSameDT=on  OutDataTypeStr=Inherit: Same as first input
  Switch : Switch  Criteria=u2 ~= 0
  ROT_CMD : Outport
  wires:
  Sum1/1 -> Gain3/1
  Gain1/1 -> Sum1/2
  Gain4/1 -> Sum1/1
  Sign/1 -> Gain4/1
  Switch/1 -> ROT_CMD/1
  Gain3/1 -> Switch/1
  Constant/1 -> Switch/3
  MOT_CMD/1 -> Gain1/1, Sign/1, Switch/2

== system Multicopter_Testbed/Visualisation/Propulsion_System/RPM_Mapping3 ==
  MOT_CMD : Inport
  Constant : Constant  Value=0
  Gain1 : Gain  DisableCoverage=on  Gain=n_max-n_min  SaturateOnIntegerOverflow=on  OutDataTypeStr=Inherit: Same as input
  Gain3 : Gain  Gain=2*pi/60
  Gain4 : Gain  DisableCoverage=on  Gain=n_min  OutDataTypeStr=Inherit: Inherit via back propagation  SaturateOnIntegerOverflow=on
  Sign : Signum  DisableCoverage=on
  Sum1 : Sum  Inputs=|++  SaturateOnIntegerOverflow=on  InputSameDT=on  OutDataTypeStr=Inherit: Same as first input
  Switch : Switch  Criteria=u2 ~= 0
  ROT_CMD : Outport
  wires:
  MOT_CMD/1 -> Switch/2, Sign/1, Gain1/1
  Constant/1 -> Switch/3
  Gain3/1 -> Switch/1
  Switch/1 -> ROT_CMD/1
  Sign/1 -> Gain4/1
  Gain4/1 -> Sum1/1
  Gain1/1 -> Sum1/2
  Sum1/1 -> Gain3/1

== system Multicopter_Testbed/Visualisation/Propulsion_System/Sliding_Average ==
  u : Inport
  Gain9 : Gain  Gain=1/100
  Sum of Elements : Sum  Inputs=+
  Tapped Delay : S-Function  FunctionName=sfix_udelay  Parameters=samptime,vinit,NumDelays,NumDelays,DelayOrder,includeCurrent,3  EnableBusSupport=off  mask(Tapped Delay Line){vinit=0.0, samptime=-1, NumDelays=99, DelayOrder=Oldest, includeCurrent=on}
      mask prompts: vinit "Simulink:masks:InitialCondition_MP"; samptime "Simulink:masks:SampleTime_MP"; NumDelays "Simulink:masks:NumberOfDelays_MP"; DelayOrder "Simulink:masks:OrderOutputVectorStartingWith_MP"; includeCurrent "Simulink:masks:IncludeCurrentInputInOutputVector_MP"
      mask help: Simulink:masks:TappedDelayLine_MD
      mask init:
      | if isempty(NumDelays)
      |    NumDelays = 1;
      | end
      mask TypeOptions DelayOrder: Simulink:masks:Oldest | Simulink:masks:Newest
      mask Display: fprintf(' %d\nDelays\n',(NumDelays))
  y : Outport
  wires:
  Tapped Delay/1 -> Sum of Elements/1
  Sum of Elements/1 -> Gain9/1
  u/1 -> Tapped Delay/1
  Gain9/1 -> y/1

== system Multicopter_Testbed/Visualisation/Propulsion_System/Sliding_Average1 ==
  u : Inport
  Gain9 : Gain  Gain=1/100
  Sum of Elements : Sum  Inputs=+
  Tapped Delay : S-Function  FunctionName=sfix_udelay  Parameters=samptime,vinit,NumDelays,NumDelays,DelayOrder,includeCurrent,3  EnableBusSupport=off  mask(Tapped Delay Line){vinit=0.0, samptime=-1, NumDelays=99, DelayOrder=Oldest, includeCurrent=on}
      mask prompts: vinit "Simulink:masks:InitialCondition_MP"; samptime "Simulink:masks:SampleTime_MP"; NumDelays "Simulink:masks:NumberOfDelays_MP"; DelayOrder "Simulink:masks:OrderOutputVectorStartingWith_MP"; includeCurrent "Simulink:masks:IncludeCurrentInputInOutputVector_MP"
      mask help: Simulink:masks:TappedDelayLine_MD
      mask init:
      | if isempty(NumDelays)
      |    NumDelays = 1;
      | end
      mask TypeOptions DelayOrder: Simulink:masks:Oldest | Simulink:masks:Newest
      mask Display: fprintf(' %d\nDelays\n',(NumDelays))
  y : Outport
  wires:
  Gain9/1 -> y/1
  u/1 -> Tapped Delay/1
  Sum of Elements/1 -> Gain9/1
  Tapped Delay/1 -> Sum of Elements/1

== system Multicopter_Testbed/Visualisation/Sensors/Compare Mix1 ==
  u1 : Inport
  u2 : Inport  Port=2
  Demux5 : Demux  Outputs=3
  Demux6 : Demux  Outputs=3
  Mux1 : Mux  Inputs=2
  Mux2 : Mux  Inputs=2
  Mux6 : Mux  Inputs=2
  y1 : Outport
  y2 : Outport  Port=2
  y3 : Outport  Port=3
  wires:
  Demux5/1 -> Mux6/2
  Demux6/1 -> Mux6/1
  u1/1 -> Demux6/1
  u2/1 -> Demux5/1
  Demux6/2 -> Mux1/1
  Demux5/2 -> Mux1/2
  Demux6/3 -> Mux2/1
  Mux6/1 -> y1/1
  Mux1/1 -> y2/1
  Mux2/1 -> y3/1
  Demux5/3 -> Mux2/2

== system Multicopter_Testbed/Visualisation/VR_View/Quad States to VR_Inputs ==
  Quad_Pos : Inport
  Quad_Att_quat : Inport  Port=2
  Viewer_Pos : Inport  Port=3
  Add : Sum  Inputs=+-
  Constant : Constant  Value=0
  Demux : Demux  Outputs=3
  Euclidean_Norm : Subsystem
      mask help: Euclidean Norm
      mask Help: Euclidean Norm
      mask Display: disp('||.||')
  Euler to VR : Subsystem  mask(Euler oritentation to VR-rotation){}
      mask help:
      | Converts a vector of euler angles to a VR-rotation.
      |
      | 1st rotation: psi   (=eul(1)) around z
      | 2nd rotation: theta (=eul(2)) around y
      | 3rd rotation: phi   (=eul(3)) around x
  Gain : Gain  Gain=-1
  Matrix Concatenate : Concatenate  NumInputs=1  Mode=Multidimensional array
  Mux : Mux  Inputs=2
  Mux1 : Mux  Inputs=3
  NED to VR-vector : Subsystem  mask(Converts NED to VR-vector){}
      mask help: [north east down] => [east up south]
  NED to VR-vector1 : Subsystem  mask(Converts NED to VR-vector){}
      mask help: [north east down] => [east up south]
  Quat to VR : Subsystem  mask(Quaternion to VR-rotation){}
      mask help: Converts a normalized quaternion to a VR-rotation.
  Scope : Scope
      settings: SaveName=ScopeData13
  Trigonometric Function : Trigonometry  Operator=atan2
  Trigonometric Function1 : Trigonometry  Operator=atan2
  VR_VW_Att : Outport
  VR_VW_Pos : Outport  Port=2
  VR_Quad_Pos : Outport  Port=3
  VR_Quad_Att : Outport  Port=4
  wires:
  Viewer_Pos/1 -> NED to VR-vector/1(ned), Add/2
  Quad_Att_quat/1 -> Quat to VR/1(q)
  Quat to VR/1(vr_rot) -> VR_Quad_Att/1
  Quad_Pos/1 -> NED to VR-vector1/1(ned), Add/1
  Add/1 -> Demux/1
  Euclidean_Norm/1(||u||) -> Trigonometric Function1/2
  Mux/1 -> Euclidean_Norm/1(u)
  Euler to VR/1(vr_rot) -> VR_VW_Att/1
  Mux1/1 -> Matrix Concatenate/1
  NED to VR-vector1/1(vr) -> Scope/1, VR_Quad_Pos/1
  NED to VR-vector/1(vr) -> VR_VW_Pos/1
  Demux/2 -> Trigonometric Function/1, Mux/2
  Demux/1 -> Trigonometric Function/2, Mux/1
  Demux/3 -> Gain/1
  Gain/1 -> Trigonometric Function1/1
  Matrix Concatenate/1 -> Euler to VR/1(euler)
  Constant/1 -> Mux1/1
  Trigonometric Function/1 -> Mux1/3
  Trigonometric Function1/1 -> Mux1/2

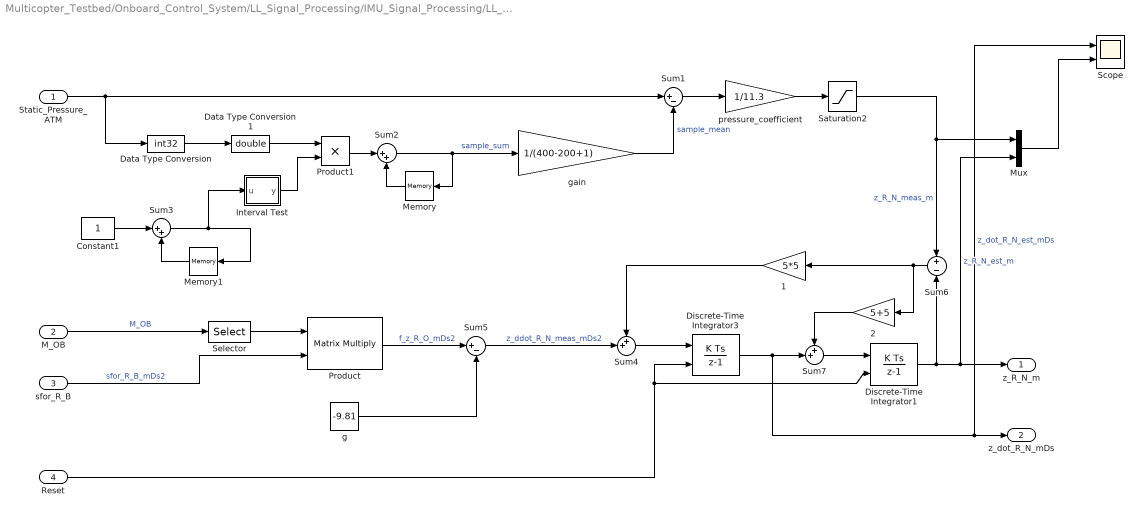
== system Multicopter_Testbed/Onboard_Control_System/LL_Signal_Processing/IMU_Signal_Processing/LL_Height_Filter ==
  Static_Pressure_ATM : Inport
  M_OB : Inport  Port=2
  sfor_R_B : Inport  Port=3
  Reset : Inport  Port=4
  1 : Gain  Gain=5*5
  2 : Gain  Gain=5+5
  Constant1 : Constant  SampleTime=0.001
  Data Type Conversion : DataTypeConversion  OutDataTypeStr=int32
  Data Type Conversion1 : DataTypeConversion  OutDataTypeStr=double
  Discrete-Time Integrator1 : DiscreteIntegrator  ExternalReset=level  SampleTime=-1  ICPrevOutput=DiscIntNeverNeededParam  ICPrevScaledInput=DiscIntNeverNeededParam
  Discrete-Time Integrator3 : DiscreteIntegrator  ExternalReset=level  SampleTime=-1  ICPrevOutput=DiscIntNeverNeededParam  ICPrevScaledInput=DiscIntNeverNeededParam
  Interval Test : Subsystem  mask(Interval Test){IntervalClosedRight=on, uplimit=400, IntervalClosedLeft=on, lowlimit=200, OutDataTypeStr=boolean}
      mask prompts: IntervalClosedRight "Simulink:masks:IntervalClosedOnRight_MP"; uplimit "Simulink:masks:UpperLimit_MP"; IntervalClosedLeft "Simulink:masks:IntervalClosedOnLeft_MP"; lowlimit "Simulink:masks:LowerLimit_MP"; OutDataTypeStr "Simulink:masks:OutputDataType_MP"
      mask help: Simulink:masks:IntervalTest_MD
      mask init:
      | if IntervalClosedLeft
      |   lOff = 0;
      |   lRelop = '<=';
      | else
      |   lOff = 0.1;
      |   lRelop = '<';
      | end
      | if IntervalClosedRight
      |   rOff = 0;
      |   uRelop = '<=';
      | else
      |   rOff = 0.1;
      |   uRelop = '<';
      | end
      | 
      | blkH = gcbh;
      | blkName = getfullname(blkH);
      | 
      | set_param([blkName,'/Upper Test'],'relop',uRelop);
      | set_param([blkName,'/Lower Test'],'relop',lRelop);
      | if strcmp(get_param(blkH,'OutDataTypeStr'),'boolean')
      | set_param([blkName,'/AND'],'OutDataTypeStr','boolean');
      | else
      | set_param([blkName,'/AND'],'OutDataTypeStr','fixdt(0, 8)');
      | end
      mask TypeOptions OutDataTypeStr: Simulink:masks:uint8 | Simulink:masks:boolean
      mask Display: plot([0 1],[0.3 0.3],[0.3 0.3],[0 1],[0 0.2 0.2],[0.35 0.35 0.55-lOff],[0.2 0.2 0.55 0.55],[0.55+lOff 0.75 0.75 0.55+rOff],[0.55 0.55 1],[0.55-rOff 0.35 0.35]);
  Memory : Memory  InheritSampleTime=on
  Memory1 : Memory  InheritSampleTime=on
  Mux : Mux  Inputs=2
  Product : Product  Multiplication=Matrix(*)  RndMeth=Zero
  Product1 : Product  RndMeth=Zero
  Saturation2 : Saturate  UpperLimit=0  LowerLimit=-500  OutDataTypeStr=double
  Scope : Scope  NumInputPorts=2
      settings: YMin=-6~-20  YMax=6~3  MaxDataPoints=5000000
  Selector : Selector  NumberOfDimensions=2  InputPortWidth=3  IndexOptions=Index vector (dialog),Select all  Indices=[3],1  OutputSizes=1,1
  Sum1 : Sum  Inputs=|+-
  Sum2 : Sum  Inputs=|++
  Sum3 : Sum  Inputs=|++  AccumDataTypeStr=int32  OutDataTypeStr=int32
  Sum4 : Sum  Inputs=++|
  Sum5 : Sum  Inputs=|+-
  Sum6 : Sum  Inputs=+|-
  Sum7 : Sum  Inputs=++|
  g : Constant  Value=-9.81  SampleTime=0.001
  gain : Gain  Gain=1/(400-200+1)
  pressure_coefficient : Gain  Gain=1/11.3
  z_R_N_m : Outport
  z_dot_R_N_mDs : Outport  Port=2
  wires:
  pressure_coefficient/1 -> Saturation2/1
  Sum1/1 -> pressure_coefficient/1
  gain/1 -> Sum1/2  "sample_mean"
  Sum2/1 -> Memory/1, gain/1  "sample_sum"
  Memory/1 -> Sum2/2
  Memory1/1 -> Sum3/2
  Constant1/1 -> Sum3/1
  Sum3/1 -> Interval Test/1(u), Memory1/1
  Static_Pressure_ATM/1 -> Data Type Conversion/1, Sum1/1
  Product1/1 -> Sum2/1
  Interval Test/1(y) -> Product1/2
  Saturation2/1 -> Sum6/1, Mux/1  "z_R_N_meas_m"
  M_OB/1 -> Selector/1  "M_OB"
  Product/1 -> Sum5/1  "f_z_R_O_mDs2"
  g/1 -> Sum5/2
  Sum5/1 -> Sum4/2  "z_ddot_R_N_meas_mDs2"
  Discrete-Time Integrator1/1 -> z_R_N_m/1, Mux/2, Sum6/2  "z_R_N_est_m"
  Sum4/1 -> Discrete-Time Integrator3/1
  Sum6/1 -> 1/1, 2/1
  1/1 -> Sum4/1
  sfor_R_B/1 -> Product/2  "sfor_R_B_mDs2"
  Selector/1 -> Product/1
  Data Type Conversion/1 -> Data Type Conversion1/1
  Data Type Conversion1/1 -> Product1/1
  Reset/1 -> Discrete-Time Integrator3/2, Discrete-Time Integrator1/2
  Discrete-Time Integrator3/1 -> Sum7/2, z_dot_R_N_mDs/1, Scope/1  "z_dot_R_N_est_mDs"
  Sum7/1 -> Discrete-Time Integrator1/1
  2/1 -> Sum7/1
  Mux/1 -> Scope/2

== system Multicopter_Testbed/Onboard_Control_System/LL_Signal_Processing/IMU_Signal_Processing/Signal_Processing1 ==
  analog : Inport
  Constant from Workspace1 : Constant  Value=Sensor.Resolution
  Data Type Conversion1 : DataTypeConversion  OutDataTypeStr=double
  Data Type Conversion4 : DataTypeConversion  OutDataTypeStr=int32
  Delay1 : Delay  DelayLength=Sensor.Latency_UNIT_s/Sampletime.Sim
  Divide1 : Product  Inputs=*/
  Product2 : Product  RndMeth=Zero
  Rate Transition : RateTransition  Integrity=off  OutPortSampleTime=Sampletime.Onboard
  Zero-Order Hold : ZeroOrderHold  SampleTime=Sensor.Sampletime
  digital : Outport
  wires:
  analog/1 -> Divide1/1
  Product2/1 -> Delay1/1
  Constant from Workspace1/1 -> Product2/2, Divide1/2
  Data Type Conversion1/1 -> Product2/1
  Data Type Conversion4/1 -> Data Type Conversion1/1
  Divide1/1 -> Data Type Conversion4/1
  Zero-Order Hold/1 -> Rate Transition/1
  Delay1/1 -> Zero-Order Hold/1
  Rate Transition/1 -> digital/1

== system Multicopter_Testbed/Onboard_Control_System/LL_Signal_Processing/IMU_Signal_Processing/Signal_Processing2 ==
  analog : Inport
  Constant from Workspace1 : Constant  Value=Sensor.Resolution
  Data Type Conversion1 : DataTypeConversion  OutDataTypeStr=double
  Data Type Conversion4 : DataTypeConversion  OutDataTypeStr=int32
  Delay1 : Delay  DelayLength=Sensor.Latency_UNIT_s/Sampletime.Sim
  Divide1 : Product  Inputs=*/
  Product2 : Product  RndMeth=Zero
  Rate Transition : RateTransition  Integrity=off  OutPortSampleTime=Sampletime.Onboard
  Zero-Order Hold : ZeroOrderHold  SampleTime=Sensor.Sampletime
  digital : Outport
  wires:
  analog/1 -> Divide1/1
  Product2/1 -> Delay1/1
  Constant from Workspace1/1 -> Product2/2, Divide1/2
  Data Type Conversion1/1 -> Product2/1
  Data Type Conversion4/1 -> Data Type Conversion1/1
  Divide1/1 -> Data Type Conversion4/1
  Zero-Order Hold/1 -> Rate Transition/1
  Delay1/1 -> Zero-Order Hold/1
  Rate Transition/1 -> digital/1

== system Multicopter_Testbed/Onboard_Control_System/LL_Signal_Processing/IMU_Signal_Processing/Signal_Processing3 ==
  analog : Inport
  Constant from Workspace1 : Constant  Value=Sensor.Resolution
  Data Type Conversion1 : DataTypeConversion  OutDataTypeStr=double
  Data Type Conversion4 : DataTypeConversion  OutDataTypeStr=int32
  Delay1 : Delay  DelayLength=Sensor.Latency_UNIT_s/Sampletime.Sim
  Divide1 : Product  Inputs=*/
  Product2 : Product  RndMeth=Zero
  Rate Transition : RateTransition  Integrity=off  OutPortSampleTime=Sampletime.Onboard
  Zero-Order Hold : ZeroOrderHold  SampleTime=Sensor.Sampletime
  digital : Outport
  wires:
  analog/1 -> Divide1/1
  Product2/1 -> Delay1/1
  Constant from Workspace1/1 -> Product2/2, Divide1/2
  Data Type Conversion1/1 -> Product2/1
  Data Type Conversion4/1 -> Data Type Conversion1/1
  Divide1/1 -> Data Type Conversion4/1
  Zero-Order Hold/1 -> Rate Transition/1
  Delay1/1 -> Zero-Order Hold/1
  Rate Transition/1 -> digital/1

== system Multicopter_Testbed/Onboard_Control_System/LL_Signal_Processing/IMU_Signal_Processing/Signal_Processing4 ==
  analog : Inport
  Constant from Workspace1 : Constant  Value=Sensor.Resolution
  Data Type Conversion1 : DataTypeConversion  OutDataTypeStr=double
  Data Type Conversion4 : DataTypeConversion  OutDataTypeStr=int32
  Delay1 : Delay  DelayLength=Sensor.Latency_UNIT_s/Sampletime.Sim
  Divide1 : Product  Inputs=*/
  Product2 : Product  RndMeth=Zero
  Rate Transition : RateTransition  Integrity=off  OutPortSampleTime=Sampletime.Onboard
  Zero-Order Hold : ZeroOrderHold  SampleTime=Sensor.Sampletime
  digital : Outport
  wires:
  analog/1 -> Divide1/1
  Product2/1 -> Delay1/1
  Constant from Workspace1/1 -> Product2/2, Divide1/2
  Data Type Conversion1/1 -> Product2/1
  Data Type Conversion4/1 -> Data Type Conversion1/1
  Divide1/1 -> Data Type Conversion4/1
  Zero-Order Hold/1 -> Rate Transition/1
  Delay1/1 -> Zero-Order Hold/1
  Rate Transition/1 -> digital/1

== system Multicopter_Testbed/Onboard_Control_System/Simulink_Control/Output_Mapping_Debug/List_Iterator ==
  Constant1 : Constant  OutDataTypeStr=int16
  Constant2 : Constant  OutDataTypeStr=int16
  Constant3 : Constant  Value=dec  OutMin=1  OutDataTypeStr=int16
  Constant4 : Constant  Value=list  OutDataTypeStr=int16
  Divide : Product  Inputs=*/  OutDataTypeStr=int16  RndMeth=Ceiling  InputSameDT=on
  FixPt Switch : Switch  Criteria=u2 > Threshold  Threshold=length(list)*dec  OutDataTypeStr=Inherit: Inherit via back propagation  ZeroCross=off  InputSameDT=on
  Index Vector : MultiPortSwitch  Inputs=1
  Sum : Sum  Inputs=++|  AccumDataTypeStr=int16  OutDataTypeStr=int16
  Unit Delay : UnitDelay  InitialCondition=1  SampleTime=-1
  index : Outport
  wires:
  Unit Delay/1 -> Sum/1, Divide/1
  FixPt Switch/1 -> Unit Delay/1
  Sum/1 -> FixPt Switch/3, FixPt Switch/2
  Constant1/1 -> FixPt Switch/1
  Constant2/1 -> Sum/2
  Constant3/1 -> Divide/2
  Constant4/1 -> Index Vector/2
  Index Vector/1 -> index/1
  Divide/1 -> Index Vector/1

== system Multicopter_Testbed/Visualisation/VR_View/Quad States to VR_Inputs/Euclidean_Norm ==
  u : Inport
  Math Function : Math  Operator=square  SaturateOnIntegerOverflow=on
  Sqrt : Sqrt  SaturateOnIntegerOverflow=on
  Sum of Elements : Sum  Inputs=+
  ||u|| : Outport
  wires:
  u/1 -> Math Function/1
  Math Function/1 -> Sum of Elements/1
  Sum of Elements/1 -> Sqrt/1
  Sqrt/1 -> ||u||/1

== system Multicopter_Testbed/Visualisation/VR_View/Quad States to VR_Inputs/Euler to VR ==
  euler : Inport
  Euler to Quat : Subsystem  mask(Euler angles to Quaternion){}
      mask help:
      | vector [phi; theta; psi] means:
      | 1. rotation: psi   (=eul(3)) around z axis
      | 2. rotation: theta (=eul(2)) around y axis
      | 3. rotation: phi   (=eul(1)) around x axis
      |
      | Regrettably implemented in Simulink
  Quat to VR : Subsystem  mask(Quaternion to VR-rotation){}
      mask help: Converts a normalized quaternion to a VR-rotation.
  Vector Concatenate1 : Concatenate  NumInputs=1  Mode=Multidimensional array
  vr_rot : Outport
  wires:
  Vector Concatenate1/1 -> Quat to VR/1(q)
  euler/1 -> Euler to Quat/1(euler)
  Euler to Quat/1(q) -> Vector Concatenate1/1
  Quat to VR/1(vr_rot) -> vr_rot/1

== system Multicopter_Testbed/Visualisation/VR_View/Quad States to VR_Inputs/NED to VR-vector ==
  ned : Inport
  Gain K*u : Gain  Gain=[0 1 0; 0 0 -1; -1 0 0]  Multiplication=Matrix(K*u)
  vr : Outport
  wires:
  ned/1 -> Gain K*u/1
  Gain K*u/1 -> vr/1

== system Multicopter_Testbed/Visualisation/VR_View/Quad States to VR_Inputs/NED to VR-vector1 ==
  ned : Inport
  Gain K*u : Gain  Gain=[0 1 0; 0 0 -1; -1 0 0]  Multiplication=Matrix(K*u)
  vr : Outport
  wires:
  ned/1 -> Gain K*u/1
  Gain K*u/1 -> vr/1
